simulink model "chap6_1sim"  (Simulink 7.0)
settings: Solver=ode45  StartTime=0.0  StopTime=30  FixedStep=0.001  RelTol=1e-3
settings Model: Creator=Administrator  LastModifiedBy=eleliuj  ExtModeTrigMode=oneshot  ExtModeArmWhenConnect=off
settings DataIOCC: LimitDataPoints=off  SignalLoggingName=sigsOut
settings OptimizationCC: BooleanDataType=off
settings DebuggingCC: SaveWithParameterizedLinksMsg=none  SignalResolutionControl=TryResolveAllWithWarning  SolverPrmCheckMsg=none  MultiTaskDSMMsg=warning  MultiTaskCondExecSysMsg=none  StrictBusMsg=None
settings HardwareCC: TargetUnknown=on
settings RTWCC: IncludeERTFirstTime=on

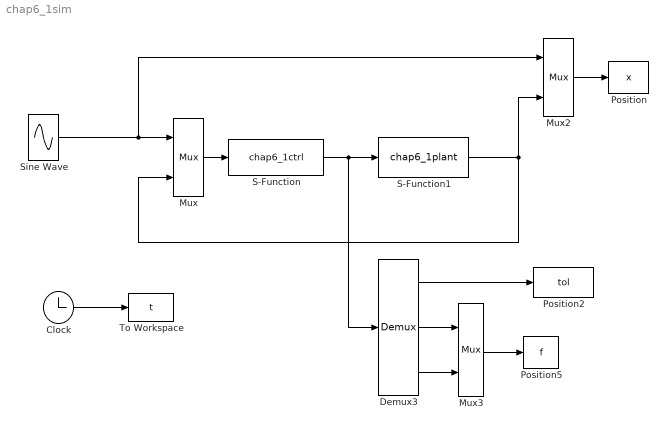
== system chap6_1sim ==
  Clock : Clock
      settings: Decimation=10
  Demux3 : Demux  Outputs=3
  Mux : Mux  Inputs=2
  Mux2 : Mux  Inputs=2
  Mux3 : Mux  Inputs=2
  Position : ToWorkspace  VariableName=x  SampleTime=-1  SaveFormat=Array
  Position2 : ToWorkspace  VariableName=tol  SampleTime=-1  SaveFormat=Array
  Position5 : ToWorkspace  VariableName=f  SampleTime=-1  SaveFormat=Array
  S-Function : S-Function  FunctionName=chap6_1ctrl
  S-Function1 : S-Function  FunctionName=chap6_1plant
  Sine Wave : Sin  SampleTime=0
  To Workspace : ToWorkspace  VariableName=t  SampleTime=-1  SaveFormat=Array
  wires:
  Mux/1 -> S-Function/1
  S-Function/1 -> S-Function1/1, Demux3/1
  S-Function1/1 -> Mux2/2, Mux/2
  Sine Wave/1 -> Mux2/1, Mux/1
  Mux3/1 -> Position5/1
  Clock/1 -> To Workspace/1
  Mux2/1 -> Position/1
  Demux3/1 -> Position2/1
  Demux3/2 -> Mux3/1
  Demux3/3 -> Mux3/2
